simulink model "windEmulatorStep3"  (R2021a)
settings: Solver=ode4  StartTime=0.0  StopTime=inf  FixedStep=0.002  RelTol=1e-3
values from neighbouring files (symbols this model uses):
  ctrlModeSpeed = logical(false)    [initStep4.m]
  ctrlModeTorque = logical(true)    [initStep4.m]
  Dm_max = 40    [initStep4.m]
  EffMechMax = 0.93    [initStep4.m]
  EffMechMin = 0.79    [initStep4.m]
  FactorEff = psi2pa*cc2m3*(1/rev2rad)    (= 0.00109733470463)    [initStep4.m]
  genMaxTorque = 0.975*acs880RatedTorque    (= 78.48165)    [initStep4.m]
  Kdamping = -500    [OptimizationResultsLoad.m]
  Kpos = 0    [OptimizationResultsLoad.m]
  nPreDrop = 2900    [initStep4.m]
  nPreDropMin = 725    [initStep4.m]
  StatusWord = bitset(StatusWord,16)    [VFD_StatusWord.m]
  T = 4    [initStep4.m]
  wheelRadius = targetWaveBotVel/targetOmega    (= 0.00477464829276)    [initStep4.m]
undefined symbols (not defined in the file or in its folder): ACS880PILimLo, ACS880PILimUp, DiscIntNeverNeededParam, Gen_REF2_Max, Gen_SpeedScaling, minPressureRef, Motor_SpeedScaling, Motor_TorqueScaling, PressureControl, ratedTorque, rpm2rps, SpeedControl, speedScalingACS800, TorqueFieldbusScale, TorqueInputControl, TorqueRefMin
libraries: fl_lib x41, nesl_utility x24, slrealtimeethercatlib x21, sh_lib x16, cstblocks x4, simulink x3, pid_lib x3, sdl_lib x1, dspstat3 x1
(part 3 of 3)

== system windEmulatorStep3/HPTOModel/ControlAlgorithm/PressureAbovePmin/SpeedControl1 ==
  ShaftSpeedMotor : Inport
  ShaftSpeedRef : Inport  Port=2
  SpeedControllerReset : Inport  Port=3
  Constant : Constant  Value=genMaxTorque
  Constant1 : Constant  Value=-genMaxTorque
  Gain2 : Gain  Gain=-1
  PID Controller : pid_lib/PID Controller  Controller=PID  Form=Parallel  TimeDomain=Discrete-time  UseExternalTs=off  SampleTime=-1  IntegratorMethod=Forward Euler  FilterMethod=Forward Euler  ControllerParametersSource=internal  P=SpeedControl.PG  I=SpeedControl.IG  D=0  UseFilter=on  N=100  TunerSelectOption=Transfer Function Based (PID Tuner App)  InitialConditionSource=internal  InitialConditionForIntegrator=0  InitialConditionForFilter=0  DifferentiatorICPrevScaledInput=0  ExternalReset=level  TrackingMode=off  Kt=1  LimitOutput=on  SatLimitsSource=external  UpperSaturationLimit=inf  LowerSaturationLimit=-inf  LinearizeAsGain=on  AntiWindupMode=none  Kb=1  POutMin=[]  POutMax=[]  IOutMin=[]  IOutMax=[]  DOutMin=[]  DOutMax=[]  NOutMin=[]  NOutMax=[]  SumOutMin=[]  SumOutMax=[]  SaturationOutMin=[]  SaturationOutMax=[]  PParamMin=[]  PParamMax=[]  IParamMin=[]  IParamMax=[]  DParamMin=[]  DParamMax=[]  NParamMin=[]  NParamMax=[]  KbParamMin=[]  KbParamMax=[]  KtParamMin=[]  KtParamMax=[]  KbOutMin=[]  KbOutMax=[]  KtOutMin=[]  KtOutMax=[]  IntegratorOutMin=[]  IntegratorOutMax=[]  FilterOutMin=[]  FilterOutMax=[]  SumI1OutMin=[]  SumI1OutMax=[]  SumI2OutMin=[]  SumI2OutMax=[]  SumI3OutMin=[]  SumI3OutMax=[]  SumI4OutMin=[]  SumI4OutMax=[]  SumDOutMin=[]  SumDOutMax=[]  DifferentiatorOutMin=[]  DifferentiatorOutMax=[]  FilterDiffOutCoefMin=[]  FilterDiffOutCoefMax=[]  ReciprocalOutMin=[]  ReciprocalOutMax=[]  SumDenOutMin=[]  SumDenOutMax=[]  SumNumOutMin=[]  SumNumOutMax=[]  DivideOutMin=[]  DivideOutMax=[]  UdiffTsProdOutMin=[]  UdiffTsProdOutMax=[]  NTsProdOutMin=[]  NTsProdOutMax=[]  UintegralTsProdOutMin=[]  UintegralTsProdOutMax=[]  UngainTsProdOutMin=[]  UngainTsProdOutMax=[]  IntegratorContinuousStateAttributes=''  IntegratorStateMustResolveToSignalObject=off  IntegratorRTWStateStorageClass=Auto  FilterContinuousStateAttributes=''  FilterStateMustResolveToSignalObject=off  FilterRTWStateStorageClass=Auto  ParallelPVariant=InternalParameters  IdealPVariant=Disabled  IVariant=InternalParameters  DVariant=InternalParameters  IntegratorVariant=Discrete  SatVariant=External  AWVariant=Passthrough  PCopyVariant=Disabled  TRVariant=Disabled  FdbkBlocksVariant=Forward  IdealPFdbkVariant=Disabled  SatFdbkVariant=Disabled  DerivativeFilterVariant=ForwardEulerFilter  NVariant=InternalParameters  NCopyVariant=Disabled  FilterICVariant=InternalICsFilter  IntegratorICVariant=InternalICs  ExternalResetVariant=ExternalReset  TRSumVariant=Passthrough  SumFdbkVariant=Disabled  SumVariant=Sum_PID  TsampFilterVariant=InternalTs  TsampNgainVariant=Passthrough  TsampIntegralVariant=Passthrough  ExternalSaturationOutDataTypeStr=Inherit: Same as second input
  Sum : Sum  Inputs=|-+
  ContolTorque : Outport
  wires:
  Gain2/1 -> ContolTorque/1  "ContolTorque"
  ShaftSpeedRef/1 -> Sum/1
  ShaftSpeedMotor/1 -> Sum/2
  Sum/1 -> PID Controller/1  "wError"
  PID Controller/1 -> Gain2/1
  SpeedControllerReset/1 -> PID Controller/2
  Constant/1 -> PID Controller/3
  Constant1/1 -> PID Controller/4

== system windEmulatorStep3/HPTOModel/ControlAlgorithm/PressureAbovePmin/TorqueControl1 ==
  TorqueRef : Inport
  Constant : Constant  Value=-1
  Constant1 : Constant
  Switch : Switch
  ControlSignal1 : Outport
  wires:
  TorqueRef/1 -> Switch/2
  Constant/1 -> Switch/1
  Constant1/1 -> Switch/3
  Switch/1 -> ControlSignal1/1

== system windEmulatorStep3/HPTOModel/ControlAlgorithm/PressureBelowPmin/PressureControl1 ==
  ActualPressure : Inport
  PressureRef : Inport  Port=2
  Add : Sum
  Discrete-Time Integrator : DiscreteIntegrator  SampleTime=-1  ICPrevOutput=DiscIntNeverNeededParam  ICPrevScaledInput=DiscIntNeverNeededParam
  Gain : Gain  Gain=PressureControl.PG
  Gain1 : Gain  Gain=PressureControl.IG
  Saturation : Saturate  UpperLimit=1  LowerLimit=-1
  Sum : Sum  Inputs=|-+
  ControlSignal2 : Outport
  wires:
  PressureRef/1 -> Sum/1
  ActualPressure/1 -> Sum/2
  Sum/1 -> Discrete-Time Integrator/1, Gain/1
  Gain/1 -> Add/1
  Discrete-Time Integrator/1 -> Gain1/1
  Gain1/1 -> Add/2
  Saturation/1 -> ControlSignal2/1
  Add/1 -> Saturation/1

== system windEmulatorStep3/HPTOModel/ControlAlgorithm/PressureBelowPmin/SpeedControl1 ==
  ShaftSpeedMotor : Inport
  ShaftSpeedRef : Inport  Port=2
  SpeedControllerReset : Inport  Port=3
  Constant : Constant  Value=genMaxTorque
  Constant1 : Constant  Value=-genMaxTorque
  Gain2 : Gain  Gain=-1
  PID Controller : pid_lib/PID Controller  Controller=PID  Form=Parallel  TimeDomain=Discrete-time  UseExternalTs=off  SampleTime=-1  IntegratorMethod=Forward Euler  FilterMethod=Forward Euler  ControllerParametersSource=internal  P=SpeedControl.PG  I=SpeedControl.IG  D=0  UseFilter=on  N=100  TunerSelectOption=Transfer Function Based (PID Tuner App)  InitialConditionSource=internal  InitialConditionForIntegrator=0  InitialConditionForFilter=0  DifferentiatorICPrevScaledInput=0  ExternalReset=level  TrackingMode=off  Kt=1  LimitOutput=on  SatLimitsSource=external  UpperSaturationLimit=inf  LowerSaturationLimit=-inf  LinearizeAsGain=on  AntiWindupMode=none  Kb=1  POutMin=[]  POutMax=[]  IOutMin=[]  IOutMax=[]  DOutMin=[]  DOutMax=[]  NOutMin=[]  NOutMax=[]  SumOutMin=[]  SumOutMax=[]  SaturationOutMin=[]  SaturationOutMax=[]  PParamMin=[]  PParamMax=[]  IParamMin=[]  IParamMax=[]  DParamMin=[]  DParamMax=[]  NParamMin=[]  NParamMax=[]  KbParamMin=[]  KbParamMax=[]  KtParamMin=[]  KtParamMax=[]  KbOutMin=[]  KbOutMax=[]  KtOutMin=[]  KtOutMax=[]  IntegratorOutMin=[]  IntegratorOutMax=[]  FilterOutMin=[]  FilterOutMax=[]  SumI1OutMin=[]  SumI1OutMax=[]  SumI2OutMin=[]  SumI2OutMax=[]  SumI3OutMin=[]  SumI3OutMax=[]  SumI4OutMin=[]  SumI4OutMax=[]  SumDOutMin=[]  SumDOutMax=[]  DifferentiatorOutMin=[]  DifferentiatorOutMax=[]  FilterDiffOutCoefMin=[]  FilterDiffOutCoefMax=[]  ReciprocalOutMin=[]  ReciprocalOutMax=[]  SumDenOutMin=[]  SumDenOutMax=[]  SumNumOutMin=[]  SumNumOutMax=[]  DivideOutMin=[]  DivideOutMax=[]  UdiffTsProdOutMin=[]  UdiffTsProdOutMax=[]  NTsProdOutMin=[]  NTsProdOutMax=[]  UintegralTsProdOutMin=[]  UintegralTsProdOutMax=[]  UngainTsProdOutMin=[]  UngainTsProdOutMax=[]  IntegratorContinuousStateAttributes=''  IntegratorStateMustResolveToSignalObject=off  IntegratorRTWStateStorageClass=Auto  FilterContinuousStateAttributes=''  FilterStateMustResolveToSignalObject=off  FilterRTWStateStorageClass=Auto  ParallelPVariant=InternalParameters  IdealPVariant=Disabled  IVariant=InternalParameters  DVariant=InternalParameters  IntegratorVariant=Discrete  SatVariant=External  AWVariant=Passthrough  PCopyVariant=Disabled  TRVariant=Disabled  FdbkBlocksVariant=Forward  IdealPFdbkVariant=Disabled  SatFdbkVariant=Disabled  DerivativeFilterVariant=ForwardEulerFilter  NVariant=InternalParameters  NCopyVariant=Disabled  FilterICVariant=InternalICsFilter  IntegratorICVariant=InternalICs  ExternalResetVariant=ExternalReset  TRSumVariant=Passthrough  SumFdbkVariant=Disabled  SumVariant=Sum_PID  TsampFilterVariant=InternalTs  TsampNgainVariant=Passthrough  TsampIntegralVariant=Passthrough  ExternalSaturationOutDataTypeStr=Inherit: Same as second input
  Sum : Sum  Inputs=|-+
  ContolTorque : Outport
  wires:
  Gain2/1 -> ContolTorque/1  "ContolTorque"
  ShaftSpeedRef/1 -> Sum/1
  ShaftSpeedMotor/1 -> Sum/2
  Sum/1 -> PID Controller/1  "wError"
  PID Controller/1 -> Gain2/1
  SpeedControllerReset/1 -> PID Controller/2
  Constant/1 -> PID Controller/3
  Constant1/1 -> PID Controller/4

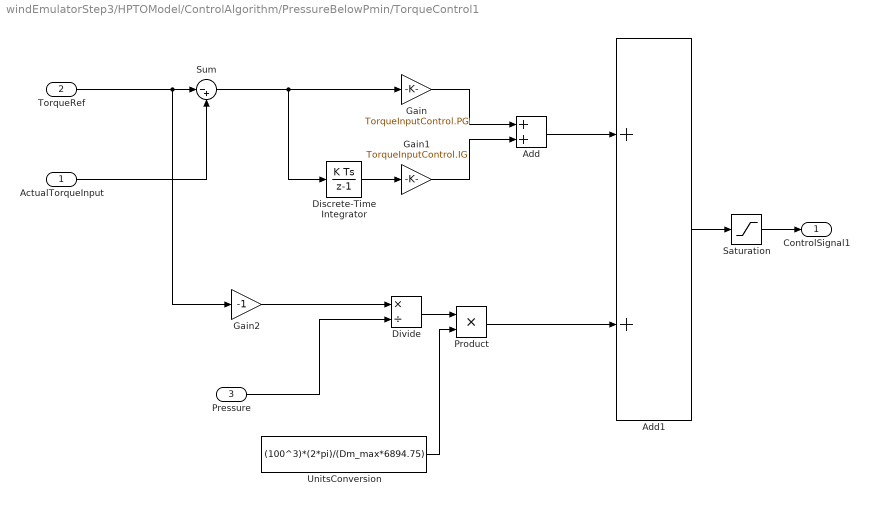
== system windEmulatorStep3/HPTOModel/ControlAlgorithm/PressureBelowPmin/TorqueControl1 ==
  ActualTorqueInput : Inport
  TorqueRef : Inport  Port=2
  Pressure : Inport  Port=3
  Add : Sum
  Add1 : Sum
  Discrete-Time Integrator : DiscreteIntegrator  SampleTime=-1  ICPrevOutput=DiscIntNeverNeededParam  ICPrevScaledInput=DiscIntNeverNeededParam
  Divide : Product  Inputs=*/
  Gain : Gain  Gain=TorqueInputControl.PG
  Gain1 : Gain  Gain=TorqueInputControl.IG
  Gain2 : Gain  Gain=-1
  Product : Product
  Saturation : Saturate  UpperLimit=1  LowerLimit=-1
  Sum : Sum  Inputs=|-+
  UnitsConversion : Constant  Value=(100^3)*(2*pi)/(Dm_max*6894.75)
  ControlSignal1 : Outport
  wires:
  ActualTorqueInput/1 -> Sum/2
  Gain/1 -> Add/1
  Discrete-Time Integrator/1 -> Gain1/1
  Sum/1 -> Discrete-Time Integrator/1, Gain/1
  TorqueRef/1 -> Gain2/1, Sum/1
  Gain1/1 -> Add/2
  Saturation/1 -> ControlSignal1/1
  Add/1 -> Add1/1
  Add1/1 -> Saturation/1
  Pressure/1 -> Divide/2
  Divide/1 -> Product/1
  Product/1 -> Add1/2
  UnitsConversion/1 -> Product/2
  Gain2/1 -> Divide/1

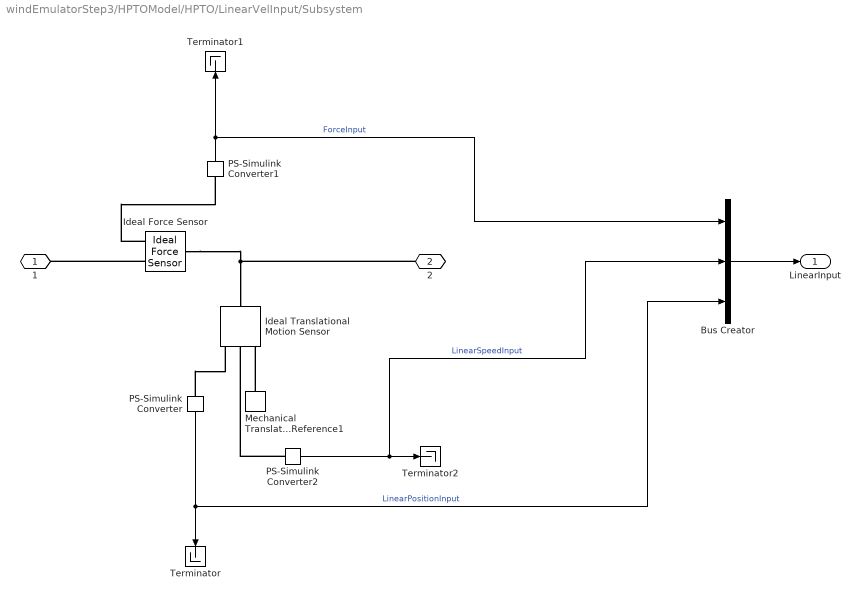
== system windEmulatorStep3/HPTOModel/HPTO/LinearVelInput/Subsystem ==
  Bus Creator : BusCreator  Inputs=3
  Ideal Force Sensor : fl_lib/Mechanical/Mechanical Sensors/Ideal Force Sensor
  Ideal Translational Motion Sensor : fl_lib/Mechanical/Mechanical Sensors/Ideal Translational Motion Sensor  offset=0 m
  Mechanical Translational Reference1 : fl_lib/Mechanical/Translational Elements/Mechanical Translational Reference
  PS-Simulink Converter : nesl_utility/PS-Simulink Converter  PhysicalDomain=network_engine_domain  SubClassName=ps_output  LeftPortType=input  RightPortType=output  PseudoPeriodic=off  Frequencies=[]  Unit=inherit  AffineConversion=off
      settings: SourceProductBaseCode=PW,SS
  PS-Simulink Converter1 : nesl_utility/PS-Simulink Converter  PhysicalDomain=network_engine_domain  SubClassName=ps_output  LeftPortType=input  RightPortType=output  PseudoPeriodic=off  Frequencies=[]  Unit=inherit  AffineConversion=off
      settings: SourceProductBaseCode=PW,SS
  PS-Simulink Converter2 : nesl_utility/PS-Simulink Converter  PhysicalDomain=network_engine_domain  SubClassName=ps_output  LeftPortType=input  RightPortType=output  PseudoPeriodic=off  Frequencies=[]  Unit=inherit  AffineConversion=off
      settings: SourceProductBaseCode=PW,SS
  Terminator : Terminator
  Terminator1 : Terminator
  Terminator2 : Terminator
  1 : PMIOPort  Side=Left
  2 : PMIOPort  Port=2  Side=Right
  LinearInput : Outport
  wires:
  PS-Simulink Converter/1 -> Terminator/1, Bus Creator/3  "LinearPositionInput"
  PS-Simulink Converter1/1 -> Bus Creator/1, Terminator1/1  "ForceInput"
  PS-Simulink Converter2/1 -> Bus Creator/2, Terminator2/1  "LinearSpeedInput"
  Bus Creator/1 -> LinearInput/1
  connections:
  Mechanical Translational Reference1/LConn1 -- Ideal Translational Motion Sensor/RConn1
  2/RConn1 -- Ideal Force Sensor/LConn1 -- Ideal Translational Motion Sensor/LConn1
  PS-Simulink Converter/LConn1 -- Ideal Translational Motion Sensor/RConn3
  PS-Simulink Converter2/LConn1 -- Ideal Translational Motion Sensor/RConn2
  Ideal Force Sensor/RConn1 -- 1/RConn1
  Ideal Force Sensor/RConn2 -- PS-Simulink Converter1/LConn1

== system windEmulatorStep3/HPTOModel/HPTO/LinearVelInput/WavebotModel ==
  PTOForce : Inport
  Fexc : Inport  Port=2
  Constant : Constant  Value=0
  Ideal Translational Velocity Source : fl_lib/Mechanical/Mechanical Sources/Ideal Translational Velocity Source
  Mechanical Translational Reference3 : fl_lib/Mechanical/Translational Elements/Mechanical Translational Reference
  Mux : Mux  Inputs=3
  Selector : Selector  InputPortWidth=3  IndexOptions=Index vector (dialog)  Indices=1  OutputSizes=1
  Simulink-PS Converter : nesl_utility/Simulink-PS Converter  PhysicalDomain=network_engine_domain  SubClassName=ps_input  LeftPortType=input  RightPortType=output  PseudoPeriodic=off  Frequencies=[]  NoiseDistribution=none  NoiseParameters=[]  Unit=1  AffineConversion=off  FilteringAndDerivatives=provide  SimscapeFilterOrder=1  InputFilterTimeConstant=0.001  UdotUserProvided=0
      settings: SourceProductBaseCode=PW,SS
  Sum : Sum  Inputs=|++
  WaveBotTF : cstblocks/LTI System  sys=Yi  IC=[]
  VelSource : PMIOPort  Side=Right
  wires:
  PTOForce/1 -> Sum/2  "PTOForce"
  Constant/1 -> Mux/3, Mux/2
  Mux/1 -> WaveBotTF/1
  WaveBotTF/1 -> Selector/1  "vel"
  Sum/1 -> Mux/1
  Selector/1 -> Simulink-PS Converter/1
  Fexc/1 -> Sum/1  "Fexc"
  connections:
  Ideal Translational Velocity Source/RConn1 -- Simulink-PS Converter/RConn1
  Mechanical Translational Reference3/LConn1 -- Ideal Translational Velocity Source/RConn2
  Ideal Translational Velocity Source/LConn1 -- VelSource/RConn1

== matlab function windEmulatorStep3/ACS880DisplayStatusWord/Parse Status Word ==
  data: StatusWord input; rdy_on output; rdy_run output; rdy_ref output; tripped output; off2 output; off3 output; swc_on_inhib output; alarm output; at_setpoint output; remote output; above_limit output; ext_ctrl_loc output; ext_run_enable output; msw_b13 output; msw_b14 output; comm_err output
function [rdy_on,rdy_run,rdy_ref,tripped,off2,off3,swc_on_inhib,alarm,...
    at_setpoint,remote,above_limit,ext_ctrl_loc,ext_run_enable,...
    msw_b13,msw_b14,comm_err]  = fcn(StatusWord)

SW = VFD_StatusWord(StatusWord);
rdy_on = SW.RDY_ON;
rdy_run = SW.RDY_RUN;
rdy_ref = SW.RDY_REF;
tripped = SW.TRIPPED;
off2 = SW.OFF_2_STA;
off3 = SW.OFF_3_STA;
swc_on_inhib = SW.SWC_ON_INHIB;
alarm = SW.ALARM;
at_setpoint = SW.AT_SETPOINT;
remote = SW.REMOTE;
above_limit = SW.ABOVE_LIMIT;
ext_ctrl_loc = SW.EXT_CTRL_LOC;
ext_run_enable = SW.EXT_RUN_ENABLE;
msw_b13 = SW.MSW_B13;
msw_b14 = SW.MSW_B14;
comm_err = SW.COMM_ERR;

== matlab function windEmulatorStep3/ACS800DisplayStatusWord/Parse Status Word ==
  data: StatusWord input; rdy_on output; rdy_run output; rdy_ref output; tripped output; off2 output; off3 output; swc_on_inhib output; alarm output; at_setpoint output; remote output; above_limit output; ext_ctrl_loc output; ext_run_enable output; msw_b13 output; msw_b14 output; comm_err output
function [rdy_on,rdy_run,rdy_ref,tripped,off2,off3,swc_on_inhib,alarm,...
    at_setpoint,remote,above_limit,ext_ctrl_loc,ext_run_enable,...
    msw_b13,msw_b14,comm_err]  = fcn(StatusWord)

SW = VFD_StatusWord(StatusWord);
rdy_on = SW.RDY_ON;
rdy_run = SW.RDY_RUN;
rdy_ref = SW.RDY_REF;
tripped = SW.TRIPPED;
off2 = SW.OFF_2_STA;
off3 = SW.OFF_3_STA;
swc_on_inhib = SW.SWC_ON_INHIB;
alarm = SW.ALARM;
at_setpoint = SW.AT_SETPOINT;
remote = SW.REMOTE;
above_limit = SW.ABOVE_LIMIT;
ext_ctrl_loc = SW.EXT_CTRL_LOC;
ext_run_enable = SW.EXT_RUN_ENABLE;
msw_b13 = SW.MSW_B13;
msw_b14 = SW.MSW_B14;
comm_err = SW.COMM_ERR;

== stateflow chart windEmulatorStep3/FexcRamp ==
  state idle
    during:
    ramp=0
    rampLast=0
  state rampup
    during:
    ramp=min(1,elapsed('sec')/rampTime)
    rampLast = ramp
  state runing
    during:
    ramp=1
    rampLast = ramp
  state rampdown
    during:
    ramp=rampLast-max(0,elapsed('sec')/rampTime)
  (default) -> idle
  rampdown -> idle : [ramp<=0]
  idle -> rampup : [runButton]
  rampup -> rampdown [order 2] : [~runButton]
  rampup -> runing [order 1] : [ramp>=1]
  runing -> rampdown : [~runButton]
  data: ramp output; runButton input; rampLast local; rampTime parameter

== stateflow chart windEmulatorStep3/ACS800FieldbusControl/ABB Fieldbus Control ==
  state UpdateStateMachine [parallel]
    during:
    swParseStatusWord();
    cwRESET = ResetFault;
    settings: executionOrder=1
    state NotReadyToOperate
      entry:
      cwOFF1_CONTROL=0;
      state ReadyToSwitchOn
        during:
        state=2
      state NotReadyToSwitchOn
        during:
        state=1
      (default) -> NotReadyToSwitchOn
      NotReadyToSwitchOn -> ReadyToSwitchOn : [swRDY_ON==1 && ...
          |  swWARNING==0 && ...
          |  EnableOperation==0]
    state initialize
      entry:
      cwInitialize();
      state=0
    state DelayOFF1
      during:
      state=5
    state ReadyToOperate
      entry:
      cwOFF1_CONTROL=1;
      state OperationDisabled
        during:
        state=3
      state OperationEnabled
        entry:
        cwENABLE_OPERATION=1;
        during:
        state=4
        exit:
        cwENABLE_OPERATION=0;
      OperationDisabled -> OperationEnabled : [swRDY_RUN==1 && ...
          |  EnableOperation==1]
      (default) -> OperationDisabled
      OperationEnabled -> OperationDisabled : [EnableOperation==0]
    initialize -> NotReadyToOperate
    (default) -> initialize
    DelayOFF1 -> NotReadyToSwitchOn : after(100,msec)
    ReadyToSwitchOn -> ReadyToOperate : [MakeReady==1 && ...
        |  swREMOTE==1]
    ReadyToOperate -> DelayOFF1 : [MakeReady==0 || ...
        |  swTRIPPED==1 || ...
        |  swSWC_ON_INHIB==1 || ...
        |  swWARNING==1]
  state UpdateControlWord [parallel]
    during:
    cwBuildControlWord();
    settings: executionOrder=2
  data: EnableOperation input; MakeReady input; swRDY_ON local; swRDY_RUN local; ResetFault input; StatusWord input; swRDY_REF local; swTRIPPED local; swOFF_2_STA local; swOFF_3_STA local; swSWC_ON_INHIB local; swAT_SETPOINT local; swEXT_RUN_ENABLE local; cwOFF2_CONTROL local; cwOFF3_CONTROL local; cwENABLE_OPERATION local; cwRAMP_OUT_ZERO local; cwRAMP_HOLD local; cwRAMP_IN_ZERO local; cwRESET local; cwREMOTE_CMD local; cwOFF1_CONTROL local; swEXT_CTRL_LOC local; swREMOTE local; ControlWord output uint16; swWARNING local; swABOVE_LIMIT local; swMSW_B13 local; swMSW_B14 local; swCOMM_ERR local; state output; cwEXT_CTRL_LOC input
  function cwInitialize:
    | function cwInitialize
    | cwOFF1_CONTROL = 0;
    | cwOFF2_CONTROL = 1;
    | cwOFF3_CONTROL = 1;
    | cwENABLE_OPERATION = 0;
    | cwRAMP_OUT_ZERO = 1;
    | cwRAMP_HOLD = 1;
    | cwRAMP_IN_ZERO = 1;
    | cwRESET = 0;
    | % cwINCHING_1 = 0;
    | % cwINCHING_2 = 0;
    | cwREMOTE_CMD = 1;
    | %cwEXT_CTRL_LOC = 0;
  function cwBuildControlWord:
    | function cwBuildControlWord
    | ControlWord = uint16(0);
    | if cwOFF1_CONTROL
    |     ControlWord = bitset(ControlWord,1);
    | end
    | if cwOFF2_CONTROL
    |     ControlWord = bitset(ControlWord,2);
    | end
    | if cwOFF3_CONTROL
    |     ControlWord = bitset(ControlWord,3);
    | end
    | if cwENABLE_OPERATION
    |     ControlWord = bitset(ControlWord,4);
    | end
    | if cwRAMP_OUT_ZERO
    |     ControlWord = bitset(ControlWord,5);
    | end
    | if cwRAMP_HOLD
    |     ControlWord = bitset(ControlWord,6);
    | end
    | if cwRAMP_IN_ZERO
    |     ControlWord = bitset(ControlWord,7);
    | end
    | if cwRESET
    |     ControlWord = bitset(ControlWord,8);
    | end
    | % if cwINCHING_1
    | %     ControlWord = bitset(ControlWord,9);
    | % end
    | % if cwINCHING_2
    | %     ControlWord = bitset(ControlWord,10);
    | % end
    | if cwREMOTE_CMD
    |     ControlWord = bitset(ControlWord,11);
    | end
    | if cwEXT_CTRL_LOC
    |     ControlWord = bitset(ControlWord,12);
    | end
  function swParseStatusWord:
    | function swParseStatusWord
    | sw = uint16(StatusWord);
    | swRDY_ON = 0;
    | swRDY_RUN = 0;
    | swRDY_REF = 0;
    | swTRIPPED = 0;
    | swOFF_2_STA = 0;
    | swOFF_3_STA = 0;
    | swSWC_ON_INHIB = 0;
    | swWARNING = 0;
    | swAT_SETPOINT = 0;
    | swREMOTE = 0;
    | swABOVE_LIMIT = 0;
    | swEXT_CTRL_LOC = 0;
    | swEXT_RUN_ENABLE = 0;
    | swMSW_B13 = 0;
    | swMSW_B14 = 0;
    | swCOMM_ERR = 0;
    | 
    | if (sw >= 2^15)
    |     swCOMM_ERR = 1;
    |     sw = sw - 2^15;
    | end
    | if (sw >= 2^14)
    |     swMSW_B14 = 1;
    |     sw = sw - 2^14;
    | end
    | if (sw >= 2^13)
    |     swMSW_B13 = 1;
    |     sw = sw - 2^13;
    | end
    | if (sw >= 2^12)
    |     swEXT_RUN_ENABLE = 1;
    |     sw = sw - 2^12;
    | end
    | if (sw >= 2^11)
    |     swEXT_CTRL_LOC = 1;
    |     sw = sw - 2^11;
    | end
    | if (sw >= 2^10)
    |     swABOVE_LIMIT = 1;
    |     sw = sw - 2^10;
    | end
    | if (sw >= 2^9)
    |     swREMOTE = 1;
    |     sw = sw - 2^9;
    | end
    | if (sw >= 2^8)
    |     swAT_SETPOINT = 1;
    |     sw = sw - 2^8;
    | end
    | if (sw >= 2^7)
    |     swWARNING = 1;
    |     sw = sw - 2^7;
    | end
    | if (sw >= 2^6)
    |     swSWC_ON_INHIB = 1;
    |     sw = sw - 2^6;
    | end
    | if (sw >= 2^5)
    |     swOFF_3_STA = 1;
    |     sw = sw - 2^5;
    | end
    | if (sw >= 2^4)
    |     swOFF_2_STA = 1;
    |     sw = sw - 2^4;
    | end
    | if (sw >= 2^3)
    |     swTRIPPED = 1;
    |     sw = sw - 2^3;
    | end
    | if (sw >= 2^2)
    |     swRDY_REF = 1;
    |     sw = sw - 2^2;
    | end
    | if (sw >= 2^1)
    |     swRDY_RUN = 1;
    |     sw = sw - 2^1;
    | end
    | if (sw >= 2^0)
    |     swRDY_ON = 1;
    |     sw = sw - 2^0;
    | end

== stateflow chart windEmulatorStep3/ACS800Ramp ==
  state idle
    during:
    ramp=0
    rampLast=0
  state rampup
    during:
    ramp=min(1,elapsed('sec')/rampTime)
    rampLast = ramp
  state runing
    during:
    ramp=1
    rampLast = ramp
  state rampdown
    during:
    ramp=rampLast-max(0,elapsed('sec')/rampTime)
  (default) -> idle
  rampdown -> idle : [ramp<=0]
  idle -> rampup : [runButton]
  rampup -> rampdown [order 2] : [~runButton]
  rampup -> runing [order 1] : [ramp>=1]
  runing -> rampdown : [~runButton]
  data: ramp output; runButton input; rampLast local; rampTime parameter

== stateflow chart windEmulatorStep3/ACS880Ramp ==
  state idle
    during:
    ramp=0
    rampLast=0
  state rampup
    during:
    ramp=min(1,elapsed('sec')/rampTime)
    rampLast = ramp
  state runing
    during:
    ramp=1
    rampLast = ramp
  state rampdown
    during:
    ramp=rampLast-max(0,elapsed('sec')/rampTime)
  (default) -> idle
  rampdown -> idle : [ramp<=0]
  idle -> rampup : [runButton]
  rampup -> rampdown [order 2] : [~runButton]
  rampup -> runing [order 1] : [ramp>=1]
  runing -> rampdown : [~runButton]
  data: ramp output; runButton input; rampLast local; rampTime parameter

== stateflow chart windEmulatorStep3/ACS880FieldbusControl/ABB Fieldbus Control ==
  state UpdateStateMachine [parallel]
    during:
    swParseStatusWord();
    cwRESET = ResetFault;
    settings: executionOrder=1
    state NotReadyToOperate
      entry:
      cwOFF1_CONTROL=0;
      state ReadyToSwitchOn
        during:
        state=2
      state NotReadyToSwitchOn
        during:
        state=1
      (default) -> NotReadyToSwitchOn
      NotReadyToSwitchOn -> ReadyToSwitchOn : [swRDY_ON==1 && ...
          |  swWARNING==0 && ...
          |  EnableOperation==0]
    state initialize
      entry:
      cwInitialize();
      state=0
    state DelayOFF1
      during:
      state=5
    state ReadyToOperate
      entry:
      cwOFF1_CONTROL=1;
      state OperationDisabled
        during:
        state=3
      state OperationEnabled
        entry:
        cwENABLE_OPERATION=1;
        during:
        state=4
        exit:
        cwENABLE_OPERATION=0;
      OperationDisabled -> OperationEnabled : [swRDY_RUN==1 && ...
          |  EnableOperation==1]
      (default) -> OperationDisabled
      OperationEnabled -> OperationDisabled : [EnableOperation==0]
    initialize -> NotReadyToOperate
    (default) -> initialize
    DelayOFF1 -> NotReadyToSwitchOn : after(100,msec)
    ReadyToSwitchOn -> ReadyToOperate : [MakeReady==1 && ...
        |  swREMOTE==1]
    ReadyToOperate -> DelayOFF1 : [MakeReady==0 || ...
        |  swTRIPPED==1 || ...
        |  swSWC_ON_INHIB==1 || ...
        |  swWARNING==1]
  state UpdateControlWord [parallel]
    during:
    cwBuildControlWord();
    settings: executionOrder=2
  data: EnableOperation input; MakeReady input; swRDY_ON local; swRDY_RUN local; ResetFault input; StatusWord input; swRDY_REF local; swTRIPPED local; swOFF_2_STA local; swOFF_3_STA local; swSWC_ON_INHIB local; swAT_SETPOINT local; swEXT_RUN_ENABLE local; cwOFF2_CONTROL local; cwOFF3_CONTROL local; cwENABLE_OPERATION local; cwRAMP_OUT_ZERO local; cwRAMP_HOLD local; cwRAMP_IN_ZERO local; cwRESET local; cwREMOTE_CMD local; cwOFF1_CONTROL local; swEXT_CTRL_LOC local; swREMOTE local; ControlWord output uint16; swWARNING local; swABOVE_LIMIT local; swMSW_B13 local; swMSW_B14 local; swCOMM_ERR local; state output; cwEXT_CTRL_LOC input
  function cwInitialize:
    | function cwInitialize
    | cwOFF1_CONTROL = 0;
    | cwOFF2_CONTROL = 1;
    | cwOFF3_CONTROL = 1;
    | cwENABLE_OPERATION = 0;
    | cwRAMP_OUT_ZERO = 1;
    | cwRAMP_HOLD = 1;
    | cwRAMP_IN_ZERO = 1;
    | cwRESET = 0;
    | % cwINCHING_1 = 0;
    | % cwINCHING_2 = 0;
    | cwREMOTE_CMD = 1;
    | %cwEXT_CTRL_LOC = 0;
  function cwBuildControlWord:
    | function cwBuildControlWord
    | ControlWord = uint16(0);
    | if cwOFF1_CONTROL
    |     ControlWord = bitset(ControlWord,1);
    | end
    | if cwOFF2_CONTROL
    |     ControlWord = bitset(ControlWord,2);
    | end
    | if cwOFF3_CONTROL
    |     ControlWord = bitset(ControlWord,3);
    | end
    | if cwENABLE_OPERATION
    |     ControlWord = bitset(ControlWord,4);
    | end
    | if cwRAMP_OUT_ZERO
    |     ControlWord = bitset(ControlWord,5);
    | end
    | if cwRAMP_HOLD
    |     ControlWord = bitset(ControlWord,6);
    | end
    | if cwRAMP_IN_ZERO
    |     ControlWord = bitset(ControlWord,7);
    | end
    | if cwRESET
    |     ControlWord = bitset(ControlWord,8);
    | end
    | % if cwINCHING_1
    | %     ControlWord = bitset(ControlWord,9);
    | % end
    | % if cwINCHING_2
    | %     ControlWord = bitset(ControlWord,10);
    | % end
    | if cwREMOTE_CMD
    |     ControlWord = bitset(ControlWord,11);
    | end
    | if cwEXT_CTRL_LOC
    |     ControlWord = bitset(ControlWord,12);
    | end
  function swParseStatusWord:
    | function swParseStatusWord
    | sw = uint16(StatusWord);
    | swRDY_ON = 0;
    | swRDY_RUN = 0;
    | swRDY_REF = 0;
    | swTRIPPED = 0;
    | swOFF_2_STA = 0;
    | swOFF_3_STA = 0;
    | swSWC_ON_INHIB = 0;
    | swWARNING = 0;
    | swAT_SETPOINT = 0;
    | swREMOTE = 0;
    | swABOVE_LIMIT = 0;
    | swEXT_CTRL_LOC = 0;
    | swEXT_RUN_ENABLE = 0;
    | swMSW_B13 = 0;
    | swMSW_B14 = 0;
    | swCOMM_ERR = 0;
    | 
    | if (sw >= 2^15)
    |     swCOMM_ERR = 1;
    |     sw = sw - 2^15;
    | end
    | if (sw >= 2^14)
    |     swMSW_B14 = 1;
    |     sw = sw - 2^14;
    | end
    | if (sw >= 2^13)
    |     swMSW_B13 = 1;
    |     sw = sw - 2^13;
    | end
    | if (sw >= 2^12)
    |     swEXT_RUN_ENABLE = 1;
    |     sw = sw - 2^12;
    | end
    | if (sw >= 2^11)
    |     swEXT_CTRL_LOC = 1;
    |     sw = sw - 2^11;
    | end
    | if (sw >= 2^10)
    |     swABOVE_LIMIT = 1;
    |     sw = sw - 2^10;
    | end
    | if (sw >= 2^9)
    |     swREMOTE = 1;
    |     sw = sw - 2^9;
    | end
    | if (sw >= 2^8)
    |     swAT_SETPOINT = 1;
    |     sw = sw - 2^8;
    | end
    | if (sw >= 2^7)
    |     swWARNING = 1;
    |     sw = sw - 2^7;
    | end
    | if (sw >= 2^6)
    |     swSWC_ON_INHIB = 1;
    |     sw = sw - 2^6;
    | end
    | if (sw >= 2^5)
    |     swOFF_3_STA = 1;
    |     sw = sw - 2^5;
    | end
    | if (sw >= 2^4)
    |     swOFF_2_STA = 1;
    |     sw = sw - 2^4;
    | end
    | if (sw >= 2^3)
    |     swTRIPPED = 1;
    |     sw = sw - 2^3;
    | end
    | if (sw >= 2^2)
    |     swRDY_REF = 1;
    |     sw = sw - 2^2;
    | end
    | if (sw >= 2^1)
    |     swRDY_RUN = 1;
    |     sw = sw - 2^1;
    | end
    | if (sw >= 2^0)
    |     swRDY_ON = 1;
    |     sw = sw - 2^0;
    | end
